simulink model "ac_sqrt"  (Simulink 9.0)
settings: Solver=FixedStepAuto  StartTime=0.0  StopTime=100  FixedStep=0.01  RelTol=1e-3
libraries: simulink x1, catapult_blocks_lib x1
settings Model: SuppressorTable=22 serialization::archive 11 0 6 0 0 0 11 0  Creator=kharer  LastModifiedBy=kharer
settings DataIOCC: SaveFormat=Dataset
settings OptimizationCC: LifeSpan=auto
settings DebuggingCC: UnderspecifiedInitializationDetection=Simplified  MergeDetectMultiDrivingBlocksExec=error  SFUnexpectedBacktrackingDiag=error  SFNoUnconditionalDefaultTransitionDiag=error  SFExecutionAtInitializationDiag=warning
settings HardwareCC: ProdBitPerPointer=64  ProdBitPerSizeT=64  ProdBitPerPtrDiffT=64  ProdLargestAtomicFloat=Float  ProdIntDivRoundTo=Zero  ProdEndianess=LittleEndian  ProdWordSize=64  ProdHWDeviceType=Intel->x86-64 (Windows64)
settings ModelReferenceCC: PropagateSignalLabelsOutOfModel=on
settings CodeAppCC: StateflowObjectComments=off
settings GRTTargetCC: TargetLangStandard=C99 (ISO)
settings ConfigComp: CovMetricSettings=dwe  CovHtmlReporting=off  CovSaveCumulativeToWorkspaceVar=off  CovSaveSingleToWorkspaceVar=off  CovExternalEMLEnable=on

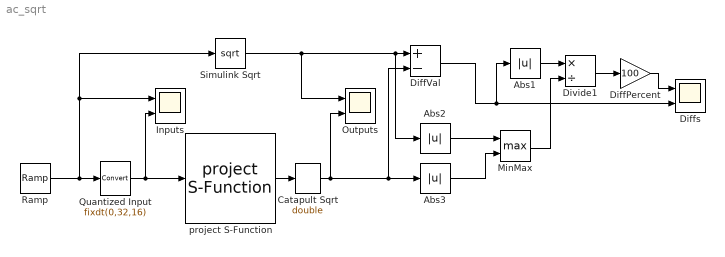
== system ac_sqrt ==
  Abs1 : Abs
  Abs2 : Abs
  Abs3 : Abs
  Catapult Sqrt : DataTypeConversion  OutDataTypeStr=double  RndMeth=Round
  DiffPercent : Gain  Gain=100
  DiffVal : Sum  Inputs=+-
  Diffs : Scope  NumInputPorts=2
  Divide1 : Product  Inputs=*/
  Inputs : Scope  NumInputPorts=2
  MinMax : MinMax  Function=max  Inputs=2
  Outputs : Scope  NumInputPorts=2
  Quantized Input : DataTypeConversion  OutDataTypeStr=fixdt(0,32,16)  RndMeth=Round
  Ramp : simulink/Sources/Ramp  slope=5  start=0  X0=0.0
  Simulink Sqrt : Sqrt  SaturateOnIntegerOverflow=on
  project S-Function : catapult_blocks_lib/project S-Function  Description=|
      | Description S-Function wrapper around the Catapult C++ function 'project'.
      | Catapult project file: '/wv/fv_engr/kevin/space/openSource/Catapult.ccs'
  wires:
  Quantized Input/1 -> project S-Function/1, Inputs/2
  Ramp/1 -> Quantized Input/1, Simulink Sqrt/1, Inputs/1
  project S-Function/1 -> Catapult Sqrt/1
  Catapult Sqrt/1 -> Abs3/1, DiffVal/2, Outputs/2
  Simulink Sqrt/1 -> Outputs/1, Abs2/1, DiffVal/1
  DiffPercent/1 -> Diffs/1
  Abs1/1 -> Divide1/1
  MinMax/1 -> Divide1/2
  Abs3/1 -> MinMax/2
  Divide1/1 -> DiffPercent/1
  Abs2/1 -> MinMax/1
  DiffVal/1 -> Abs1/1, Diffs/2
